simulink library "MedusaPremix"  (R2022b)
settings: Solver=VariableStepAuto  StartTime=0.0  StopTime=10.0  RelTol=1e-3
values from neighbouring files (symbols this model uses):
  PremixConfig = struct('sample_rate_in_hertz', sample_rate_in_hertz,                            'frame_size', frame_size,                            'rgain_SILENT_GAIN', rgain_SILENT_GAIN,                            'granularity', internal_granularity,                            'LR_in', LR_in, 'LR_out', LR_out,                            'CS_in', CS_in, 'CS_out', CS_out,                            'NumCenterOut' ...(+550 chars)    [MedusaPremixInit.m]
  PremixTune = MedusaPremixTuneInit(tuneFileName, headrestTuneFileName, overheadTuneFileName, MedusaParams)    [MedusaPremixInit.m]    (also in MedusaPremixTuneInit.m = load(tuneFileName))
undefined symbols (not defined in the file or in its folder): carModel, mode, MSConfig, Row
libraries: TuneVar x286, TOP x202, dspmtrx3 x146, FeaturePath x86, matrix_library x20, PooliirLib x8, Pooliir x4
(part 13 of 22)

== system MedusaPremix/Premix51/Full Mixing Matrix_Center Surround/Fader Downmix/Fading Forward ==
  backFadeGain : Inport
  forwardDownmixThreshold : Inport  Port=2
  forwardDownmixMax : Inport  Port=3
  Action Port : ActionPort
  Constant : Constant  OutDataTypeStr=single
  Divide : Product  Inputs=*/
  EPS : Constant  Value=eps('single')
  Max : MinMax  Function=max  Inputs=2
  Min : MinMax  Inputs=2
  Multiply : Product
  Subtract : Sum  Inputs=+-
  downmix : Outport  VectorParamsAs1DForOutWhenUnconnected=off
  wires:
  backFadeGain/1 -> Min/1
  forwardDownmixThreshold/1 -> Min/2, Max/1
  Constant/1 -> Subtract/1
  EPS/1 -> Max/2
  Min/1 -> Divide/1  "minFadeGain"
  Max/1 -> Divide/2
  Divide/1 -> Subtract/2
  Subtract/1 -> Multiply/1
  forwardDownmixMax/1 -> Multiply/2
  Multiply/1 -> downmix/1

== system MedusaPremix/Premix51/Full Mixing Matrix_Center Surround/Surround Level Control/Ramper ==
  RTC Recv Trigger : Inport
  target gains (linear) : Inport  Port=2
  ramp rate : Inport  Port=3
  ramp time : Inport  Port=4
  check sequence trigger : Inport  Port=5
  Data Store Memory : DataStoreMemory  DataStoreName=Premix_Freeze_CS  ReadBeforeWriteMsg=warning  WriteAfterWriteMsg=warning  WriteAfterReadMsg=warning  ShowAdditionalParam=off  OutDataTypeStr=boolean
  Data Store Memory1 : DataStoreMemory  DataStoreName=Premix_frameCount_CS  ReadBeforeWriteMsg=warning  WriteAfterWriteMsg=warning  WriteAfterReadMsg=warning  InitialValue=zeros(MedusaPremixConfig.CS_out,MedusaPremixConfig.CS_in)  ShowAdditionalParam=off  OutDataTypeStr=int32
  Data Store Memory2 : DataStoreMemory  DataStoreName=Premix_rampCoeff_CS  ReadBeforeWriteMsg=warning  WriteAfterWriteMsg=warning  WriteAfterReadMsg=warning  InitialValue=ones(MedusaPremixConfig.CS_out,MedusaPremixConfig.CS_in)  ShowAdditionalParam=off  OutDataTypeStr=single
  check sequence : MATLAB Function  TreatAsAtomicUnit=on
  control : MATLAB Function  TreatAsAtomicUnit=on
  process : MATLAB Function  TreatAsAtomicUnit=on
  ramping done : Outport  VectorParamsAs1DForOutWhenUnconnected=off
  wires:
  ramp time/1 -> control/3(rampTime)
  ramp rate/1 -> control/2(rampRate)
  check sequence trigger/1 -> check sequence/Trigger
  check sequence/1(done) -> ramping done/1
  RTC Recv Trigger/1 -> control/Trigger
  target gains (linear)/1 -> control/1(target_gains_linear)

== system MedusaPremix/Premix51/Full Mixing Matrix_Left/Fader Downmix/Fading Backward ==
  frontFadeGain : Inport
  backwardDownmixThreshold : Inport  Port=2
  backwardDownmixMax : Inport  Port=3
  Action Port : ActionPort
  Constant : Constant  OutDataTypeStr=single
  Divide : Product  Inputs=*/
  EPS : Constant  Value=eps('single')
  Max : MinMax  Function=max  Inputs=2
  Min : MinMax  Inputs=2
  Multiply : Product
  Subtract : Sum  Inputs=+-
  downmix : Outport  VectorParamsAs1DForOutWhenUnconnected=off
  wires:
  frontFadeGain/1 -> Min/1
  backwardDownmixThreshold/1 -> Min/2, Max/1
  Constant/1 -> Subtract/1
  EPS/1 -> Max/2
  Min/1 -> Divide/1  "minFadeGain"
  Max/1 -> Divide/2
  Divide/1 -> Subtract/2
  Subtract/1 -> Multiply/1
  backwardDownmixMax/1 -> Multiply/2
  Multiply/1 -> downmix/1

== system MedusaPremix/Premix51/Full Mixing Matrix_Left/Fader Downmix/Fading Forward ==
  backFadeGain : Inport
  forwardDownmixThreshold : Inport  Port=2
  forwardDownmixMax : Inport  Port=3
  Action Port : ActionPort
  Constant : Constant  OutDataTypeStr=single
  Divide : Product  Inputs=*/
  EPS : Constant  Value=eps('single')
  Max : MinMax  Function=max  Inputs=2
  Min : MinMax  Inputs=2
  Multiply : Product
  Subtract : Sum  Inputs=+-
  downmix : Outport  VectorParamsAs1DForOutWhenUnconnected=off
  wires:
  backFadeGain/1 -> Min/1
  forwardDownmixThreshold/1 -> Min/2, Max/1
  Constant/1 -> Subtract/1
  EPS/1 -> Max/2
  Min/1 -> Divide/1  "minFadeGain"
  Max/1 -> Divide/2
  Divide/1 -> Subtract/2
  Subtract/1 -> Multiply/1
  forwardDownmixMax/1 -> Multiply/2
  Multiply/1 -> downmix/1

== system MedusaPremix/Premix51/Full Mixing Matrix_Left/Surround Level Control/Ramper ==
  RTC Recv Trigger : Inport
  target gains (linear) : Inport  Port=2
  ramp rate : Inport  Port=3
  ramp time : Inport  Port=4
  check sequence trigger : Inport  Port=5
  Data Store Memory : DataStoreMemory  DataStoreName=Premix_Freeze_Left  ReadBeforeWriteMsg=warning  WriteAfterWriteMsg=warning  WriteAfterReadMsg=warning  ShowAdditionalParam=off  OutDataTypeStr=boolean
  Data Store Memory1 : DataStoreMemory  DataStoreName=Premix_frameCount_Left  ReadBeforeWriteMsg=warning  WriteAfterWriteMsg=warning  WriteAfterReadMsg=warning  InitialValue=zeros(MedusaPremixConfig.LR_out,MedusaPremixConfig.LR_in)  ShowAdditionalParam=off  OutDataTypeStr=int32
  Data Store Memory2 : DataStoreMemory  DataStoreName=Premix_rampCoeff_Left  ReadBeforeWriteMsg=warning  WriteAfterWriteMsg=warning  WriteAfterReadMsg=warning  InitialValue=ones(MedusaPremixConfig.LR_out,MedusaPremixConfig.LR_in)  ShowAdditionalParam=off  OutDataTypeStr=single
  check sequence : MATLAB Function  TreatAsAtomicUnit=on
  control : MATLAB Function  TreatAsAtomicUnit=on
  process : MATLAB Function  TreatAsAtomicUnit=on
  ramping done : Outport  VectorParamsAs1DForOutWhenUnconnected=off
  wires:
  ramp time/1 -> control/3(rampTime)
  ramp rate/1 -> control/2(rampRate)
  check sequence trigger/1 -> check sequence/Trigger
  check sequence/1(done) -> ramping done/1
  RTC Recv Trigger/1 -> control/Trigger
  target gains (linear)/1 -> control/1(target_gains_linear)

== system MedusaPremix/Premix51/Full Mixing Matrix_Right/Fader Downmix/Fading Backward ==
  frontFadeGain : Inport
  backwardDownmixThreshold : Inport  Port=2
  backwardDownmixMax : Inport  Port=3
  Action Port : ActionPort
  Constant : Constant  OutDataTypeStr=single
  Divide : Product  Inputs=*/
  EPS : Constant  Value=eps('single')
  Max : MinMax  Function=max  Inputs=2
  Min : MinMax  Inputs=2
  Multiply : Product
  Subtract : Sum  Inputs=+-
  downmix : Outport  VectorParamsAs1DForOutWhenUnconnected=off
  wires:
  frontFadeGain/1 -> Min/1
  backwardDownmixThreshold/1 -> Min/2, Max/1
  Constant/1 -> Subtract/1
  EPS/1 -> Max/2
  Min/1 -> Divide/1  "minFadeGain"
  Max/1 -> Divide/2
  Divide/1 -> Subtract/2
  Subtract/1 -> Multiply/1
  backwardDownmixMax/1 -> Multiply/2
  Multiply/1 -> downmix/1

== system MedusaPremix/Premix51/Full Mixing Matrix_Right/Fader Downmix/Fading Forward ==
  backFadeGain : Inport
  forwardDownmixThreshold : Inport  Port=2
  forwardDownmixMax : Inport  Port=3
  Action Port : ActionPort
  Constant : Constant  OutDataTypeStr=single
  Divide : Product  Inputs=*/
  EPS : Constant  Value=eps('single')
  Max : MinMax  Function=max  Inputs=2
  Min : MinMax  Inputs=2
  Multiply : Product
  Subtract : Sum  Inputs=+-
  downmix : Outport  VectorParamsAs1DForOutWhenUnconnected=off
  wires:
  backFadeGain/1 -> Min/1
  forwardDownmixThreshold/1 -> Min/2, Max/1
  Constant/1 -> Subtract/1
  EPS/1 -> Max/2
  Min/1 -> Divide/1  "minFadeGain"
  Max/1 -> Divide/2
  Divide/1 -> Subtract/2
  Subtract/1 -> Multiply/1
  forwardDownmixMax/1 -> Multiply/2
  Multiply/1 -> downmix/1

== system MedusaPremix/Premix51/Full Mixing Matrix_Right/Surround Level Control/Ramper ==
  RTC Recv Trigger : Inport
  target gains (linear) : Inport  Port=2
  ramp rate : Inport  Port=3
  ramp time : Inport  Port=4
  check sequence trigger : Inport  Port=5
  Data Store Memory : DataStoreMemory  DataStoreName=Premix_Freeze_Right  ReadBeforeWriteMsg=warning  WriteAfterWriteMsg=warning  WriteAfterReadMsg=warning  ShowAdditionalParam=off  OutDataTypeStr=boolean
  Data Store Memory1 : DataStoreMemory  DataStoreName=Premix_frameCount_Right  ReadBeforeWriteMsg=warning  WriteAfterWriteMsg=warning  WriteAfterReadMsg=warning  InitialValue=zeros(MedusaPremixConfig.LR_out,MedusaPremixConfig.LR_in)  ShowAdditionalParam=off  OutDataTypeStr=int32
  Data Store Memory2 : DataStoreMemory  DataStoreName=Premix_rampCoeff_Right  ReadBeforeWriteMsg=warning  WriteAfterWriteMsg=warning  WriteAfterReadMsg=warning  InitialValue=ones(MedusaPremixConfig.LR_out,MedusaPremixConfig.LR_in)  ShowAdditionalParam=off  OutDataTypeStr=single
  check sequence : MATLAB Function  TreatAsAtomicUnit=on
  control : MATLAB Function  TreatAsAtomicUnit=on
  process : MATLAB Function  TreatAsAtomicUnit=on
  ramping done : Outport  VectorParamsAs1DForOutWhenUnconnected=off
  wires:
  ramp time/1 -> control/3(rampTime)
  ramp rate/1 -> control/2(rampRate)
  check sequence trigger/1 -> check sequence/Trigger
  check sequence/1(done) -> ramping done/1
  RTC Recv Trigger/1 -> control/Trigger
  target gains (linear)/1 -> control/1(target_gains_linear)

== system MedusaPremix/Premix51WithMonoSurround/CS Processing/Mono-Surround/Left Mixer ==
  AudioIn : Inport
  MixCoeff : Inport  Port=2
  Matrix Multiply1 : Product  Multiplication=Matrix(*)
  Transpose1 : Math  Operator=transpose  SignedPower=on
  Output : Outport  VectorParamsAs1DForOutWhenUnconnected=off
  wires:
  Matrix Multiply1/1 -> Output/1
  AudioIn/1 -> Matrix Multiply1/1
  MixCoeff/1 -> Transpose1/1
  Transpose1/1 -> Matrix Multiply1/2

== system MedusaPremix/Premix51WithMonoSurround/CS Processing/Mono-Surround/MS Tune ==
  TOP : TOP/TOP  TriggerInit=[260 -150 405 -90]  TopName=Phi  DataType=single  BankNumber=0  Role=Automatic
      settings: SourceProductName=Bose Talaria
  TOP1 : TOP/TOP  TriggerInit=[260 -70 405 -10]  TopName=CosPhi  DataType=single  BankNumber=0  Role=Automatic
      settings: SourceProductName=Bose Talaria
  TOP2 : TOP/TOP  TriggerInit=[260 10 405 70]  TopName=SinPhi  DataType=single  BankNumber=0  Role=Automatic
      settings: SourceProductName=Bose Talaria
  TranslateTrigger : TuneVar/TranslateTrigger  TriggerInit=[66 -245 104 -190]
      settings: SourceProductName=Bose Talaria
  Tune Variable : TuneVar/Tune Variable  TuneName=PhaseAngle  SpecifyMaxSize=off  VariableDim=1 (Row)  MaxSize=[1 1]  PackageName=mode  TunabilityNumber=1  MinValue=[]  MaxValue=[]  TriggerInit=[-270 -65 -100 -15]  MaskValue=MSConfig.DefaultPhaseAngle
      settings: SourceProductName=Bose Talaria
  translation : MATLAB Function  TreatAsAtomicUnit=on
  phi : Outport  VectorParamsAs1DForOutWhenUnconnected=off
  cos(phi) : Outport  Port=2  VectorParamsAs1DForOutWhenUnconnected=off
  sin(phi) : Outport  Port=3  VectorParamsAs1DForOutWhenUnconnected=off
  wires:
  translation/1(phi) -> TOP/1
  TranslateTrigger/1 -> translation/Trigger
  TOP/1 -> phi/1  "Phi"
  Tune Variable/1 -> translation/1(PhaseAngle)  "PhaseAngle"
  translation/2(cos_phi) -> TOP1/1
  TOP1/1 -> cos(phi)/1  "CosPhi"
  translation/3(sin_phi) -> TOP2/1
  TOP2/1 -> sin(phi)/1  "SinPhi"

== system MedusaPremix/Premix51WithMonoSurround/CS Processing/Mono-Surround/Right Mixer ==
  AudioIn : Inport
  MixCoeff : Inport  Port=2
  Matrix Multiply1 : Product  Multiplication=Matrix(*)
  Transpose1 : Math  Operator=transpose  SignedPower=on
  Output : Outport  VectorParamsAs1DForOutWhenUnconnected=off
  wires:
  Matrix Multiply1/1 -> Output/1
  AudioIn/1 -> Matrix Multiply1/1
  MixCoeff/1 -> Transpose1/1
  Transpose1/1 -> Matrix Multiply1/2

== system MedusaPremix/Premix51WithMonoSurround/CS Processing/Mono-Surround/Right Mixer1 ==
  AudioIn : Inport
  MixCoeff : Inport  Port=2
  Matrix Multiply1 : Product  Multiplication=Matrix(*)
  Transpose1 : Math  Operator=transpose  SignedPower=on
  Output : Outport  VectorParamsAs1DForOutWhenUnconnected=off
  wires:
  Matrix Multiply1/1 -> Output/1
  AudioIn/1 -> Matrix Multiply1/1
  MixCoeff/1 -> Transpose1/1
  Transpose1/1 -> Matrix Multiply1/2

== system MedusaPremix/Premix51WithMonoSurround/CS Processing/Mono-Surround/SOS A ==
  AudioIn : Inport
  TuneIn : Inport  Port=2
  Hilbert SOS A : Subsystem  TreatAsAtomicUnit=on
  If : If  IfExpression=(u1==0) | (u1==180)
  Merge : Merge
  Pass-through : Subsystem  TreatAsAtomicUnit=on
  Out : Outport  VectorParamsAs1DForOutWhenUnconnected=off
  wires:
  AudioIn/1 -> Hilbert SOS A/1(AudioIn), Pass-through/1(In1)
  If/1 -> Pass-through/Action
  If/2 -> Hilbert SOS A/Action
  TuneIn/1 -> If/1
  Pass-through/1(Out1) -> Merge/1
  Hilbert SOS A/1(Out) -> Merge/2
  Merge/1 -> Out/1

== system MedusaPremix/Premix51WithMonoSurround/CS Processing/Mono-Surround/SOS B ==
  AudioIn : Inport
  TuneIn : Inport  Port=2
  Hilbert SOS B : Subsystem  TreatAsAtomicUnit=on
  If : If  IfExpression=(u1==0) | (u1==180)
  Merge : Merge
  Pass-through : Subsystem  TreatAsAtomicUnit=on
  Out : Outport  VectorParamsAs1DForOutWhenUnconnected=off
  wires:
  AudioIn/1 -> Hilbert SOS B/1(AudioIn), Pass-through/1(In1)
  If/1 -> Pass-through/Action
  If/2 -> Hilbert SOS B/Action
  TuneIn/1 -> If/1
  Pass-through/1(Out1) -> Merge/1
  Hilbert SOS B/1(Out) -> Merge/2
  Merge/1 -> Out/1

== system MedusaPremix/Premix51WithMonoSurround/Full Mixing Matrix_Center Surround/Fader Downmix/Fading Backward ==
  frontFadeGain : Inport
  backwardDownmixThreshold : Inport  Port=2
  backwardDownmixMax : Inport  Port=3
  Action Port : ActionPort
  Constant : Constant  OutDataTypeStr=single
  Divide : Product  Inputs=*/
  EPS : Constant  Value=eps('single')
  Max : MinMax  Function=max  Inputs=2
  Min : MinMax  Inputs=2
  Multiply : Product
  Subtract : Sum  Inputs=+-
  downmix : Outport  VectorParamsAs1DForOutWhenUnconnected=off
  wires:
  frontFadeGain/1 -> Min/1
  backwardDownmixThreshold/1 -> Min/2, Max/1
  Constant/1 -> Subtract/1
  EPS/1 -> Max/2
  Min/1 -> Divide/1  "minFadeGain"
  Max/1 -> Divide/2
  Divide/1 -> Subtract/2
  Subtract/1 -> Multiply/1
  backwardDownmixMax/1 -> Multiply/2
  Multiply/1 -> downmix/1

== system MedusaPremix/Premix51WithMonoSurround/Full Mixing Matrix_Center Surround/Fader Downmix/Fading Forward ==
  backFadeGain : Inport
  forwardDownmixThreshold : Inport  Port=2
  forwardDownmixMax : Inport  Port=3
  Action Port : ActionPort
  Constant : Constant  OutDataTypeStr=single
  Divide : Product  Inputs=*/
  EPS : Constant  Value=eps('single')
  Max : MinMax  Function=max  Inputs=2
  Min : MinMax  Inputs=2
  Multiply : Product
  Subtract : Sum  Inputs=+-
  downmix : Outport  VectorParamsAs1DForOutWhenUnconnected=off
  wires:
  backFadeGain/1 -> Min/1
  forwardDownmixThreshold/1 -> Min/2, Max/1
  Constant/1 -> Subtract/1
  EPS/1 -> Max/2
  Min/1 -> Divide/1  "minFadeGain"
  Max/1 -> Divide/2
  Divide/1 -> Subtract/2
  Subtract/1 -> Multiply/1
  forwardDownmixMax/1 -> Multiply/2
  Multiply/1 -> downmix/1

== system MedusaPremix/Premix51WithMonoSurround/Full Mixing Matrix_Center Surround/Surround Level Control/Ramper ==
  RTC Recv Trigger : Inport
  target gains (linear) : Inport  Port=2
  ramp rate : Inport  Port=3
  ramp time : Inport  Port=4
  check sequence trigger : Inport  Port=5
  Data Store Memory : DataStoreMemory  DataStoreName=Premix_Freeze_CS  ReadBeforeWriteMsg=warning  WriteAfterWriteMsg=warning  WriteAfterReadMsg=warning  ShowAdditionalParam=off  OutDataTypeStr=boolean
  Data Store Memory1 : DataStoreMemory  DataStoreName=Premix_frameCount_CS  ReadBeforeWriteMsg=warning  WriteAfterWriteMsg=warning  WriteAfterReadMsg=warning  InitialValue=zeros(MedusaPremixConfig.CS_out,MedusaPremixConfig.CS_in)  ShowAdditionalParam=off  OutDataTypeStr=int32
  Data Store Memory2 : DataStoreMemory  DataStoreName=Premix_rampCoeff_CS  ReadBeforeWriteMsg=warning  WriteAfterWriteMsg=warning  WriteAfterReadMsg=warning  InitialValue=ones(MedusaPremixConfig.CS_out,MedusaPremixConfig.CS_in)  ShowAdditionalParam=off  OutDataTypeStr=single
  check sequence : MATLAB Function  TreatAsAtomicUnit=on
  control : MATLAB Function  TreatAsAtomicUnit=on
  process : MATLAB Function  TreatAsAtomicUnit=on
  ramping done : Outport  VectorParamsAs1DForOutWhenUnconnected=off
  wires:
  ramp time/1 -> control/3(rampTime)
  ramp rate/1 -> control/2(rampRate)
  check sequence trigger/1 -> check sequence/Trigger
  check sequence/1(done) -> ramping done/1
  RTC Recv Trigger/1 -> control/Trigger
  target gains (linear)/1 -> control/1(target_gains_linear)

== system MedusaPremix/Premix51WithMonoSurround/Full Mixing Matrix_Left/Fader Downmix/Fading Backward ==
  frontFadeGain : Inport
  backwardDownmixThreshold : Inport  Port=2
  backwardDownmixMax : Inport  Port=3
  Action Port : ActionPort
  Constant : Constant  OutDataTypeStr=single
  Divide : Product  Inputs=*/
  EPS : Constant  Value=eps('single')
  Max : MinMax  Function=max  Inputs=2
  Min : MinMax  Inputs=2
  Multiply : Product
  Subtract : Sum  Inputs=+-
  downmix : Outport  VectorParamsAs1DForOutWhenUnconnected=off
  wires:
  frontFadeGain/1 -> Min/1
  backwardDownmixThreshold/1 -> Min/2, Max/1
  Constant/1 -> Subtract/1
  EPS/1 -> Max/2
  Min/1 -> Divide/1  "minFadeGain"
  Max/1 -> Divide/2
  Divide/1 -> Subtract/2
  Subtract/1 -> Multiply/1
  backwardDownmixMax/1 -> Multiply/2
  Multiply/1 -> downmix/1

== system MedusaPremix/Premix51WithMonoSurround/Full Mixing Matrix_Left/Fader Downmix/Fading Forward ==
  backFadeGain : Inport
  forwardDownmixThreshold : Inport  Port=2
  forwardDownmixMax : Inport  Port=3
  Action Port : ActionPort
  Constant : Constant  OutDataTypeStr=single
  Divide : Product  Inputs=*/
  EPS : Constant  Value=eps('single')
  Max : MinMax  Function=max  Inputs=2
  Min : MinMax  Inputs=2
  Multiply : Product
  Subtract : Sum  Inputs=+-
  downmix : Outport  VectorParamsAs1DForOutWhenUnconnected=off
  wires:
  backFadeGain/1 -> Min/1
  forwardDownmixThreshold/1 -> Min/2, Max/1
  Constant/1 -> Subtract/1
  EPS/1 -> Max/2
  Min/1 -> Divide/1  "minFadeGain"
  Max/1 -> Divide/2
  Divide/1 -> Subtract/2
  Subtract/1 -> Multiply/1
  forwardDownmixMax/1 -> Multiply/2
  Multiply/1 -> downmix/1

== system MedusaPremix/Premix51WithMonoSurround/Full Mixing Matrix_Left/Surround Level Control/Ramper ==
  RTC Recv Trigger : Inport
  target gains (linear) : Inport  Port=2
  ramp rate : Inport  Port=3
  ramp time : Inport  Port=4
  check sequence trigger : Inport  Port=5
  Data Store Memory : DataStoreMemory  DataStoreName=Premix_Freeze_Left  ReadBeforeWriteMsg=warning  WriteAfterWriteMsg=warning  WriteAfterReadMsg=warning  ShowAdditionalParam=off  OutDataTypeStr=boolean
  Data Store Memory1 : DataStoreMemory  DataStoreName=Premix_frameCount_Left  ReadBeforeWriteMsg=warning  WriteAfterWriteMsg=warning  WriteAfterReadMsg=warning  InitialValue=zeros(MedusaPremixConfig.LR_out,MedusaPremixConfig.LR_in)  ShowAdditionalParam=off  OutDataTypeStr=int32
  Data Store Memory2 : DataStoreMemory  DataStoreName=Premix_rampCoeff_Left  ReadBeforeWriteMsg=warning  WriteAfterWriteMsg=warning  WriteAfterReadMsg=warning  InitialValue=ones(MedusaPremixConfig.LR_out,MedusaPremixConfig.LR_in)  ShowAdditionalParam=off  OutDataTypeStr=single
  check sequence : MATLAB Function  TreatAsAtomicUnit=on
  control : MATLAB Function  TreatAsAtomicUnit=on
  process : MATLAB Function  TreatAsAtomicUnit=on
  ramping done : Outport  VectorParamsAs1DForOutWhenUnconnected=off
  wires:
  ramp time/1 -> control/3(rampTime)
  ramp rate/1 -> control/2(rampRate)
  check sequence trigger/1 -> check sequence/Trigger
  check sequence/1(done) -> ramping done/1
  RTC Recv Trigger/1 -> control/Trigger
  target gains (linear)/1 -> control/1(target_gains_linear)

== system MedusaPremix/Premix51WithMonoSurround/Full Mixing Matrix_Right/Fader Downmix/Fading Backward ==
  frontFadeGain : Inport
  backwardDownmixThreshold : Inport  Port=2
  backwardDownmixMax : Inport  Port=3
  Action Port : ActionPort
  Constant : Constant  OutDataTypeStr=single
  Divide : Product  Inputs=*/
  EPS : Constant  Value=eps('single')
  Max : MinMax  Function=max  Inputs=2
  Min : MinMax  Inputs=2
  Multiply : Product
  Subtract : Sum  Inputs=+-
  downmix : Outport  VectorParamsAs1DForOutWhenUnconnected=off
  wires:
  frontFadeGain/1 -> Min/1
  backwardDownmixThreshold/1 -> Min/2, Max/1
  Constant/1 -> Subtract/1
  EPS/1 -> Max/2
  Min/1 -> Divide/1  "minFadeGain"
  Max/1 -> Divide/2
  Divide/1 -> Subtract/2
  Subtract/1 -> Multiply/1
  backwardDownmixMax/1 -> Multiply/2
  Multiply/1 -> downmix/1

== system MedusaPremix/Premix51WithMonoSurround/Full Mixing Matrix_Right/Fader Downmix/Fading Forward ==
  backFadeGain : Inport
  forwardDownmixThreshold : Inport  Port=2
  forwardDownmixMax : Inport  Port=3
  Action Port : ActionPort
  Constant : Constant  OutDataTypeStr=single
  Divide : Product  Inputs=*/
  EPS : Constant  Value=eps('single')
  Max : MinMax  Function=max  Inputs=2
  Min : MinMax  Inputs=2
  Multiply : Product
  Subtract : Sum  Inputs=+-
  downmix : Outport  VectorParamsAs1DForOutWhenUnconnected=off
  wires:
  backFadeGain/1 -> Min/1
  forwardDownmixThreshold/1 -> Min/2, Max/1
  Constant/1 -> Subtract/1
  EPS/1 -> Max/2
  Min/1 -> Divide/1  "minFadeGain"
  Max/1 -> Divide/2
  Divide/1 -> Subtract/2
  Subtract/1 -> Multiply/1
  forwardDownmixMax/1 -> Multiply/2
  Multiply/1 -> downmix/1

== system MedusaPremix/Premix51WithMonoSurround/Full Mixing Matrix_Right/Surround Level Control/Ramper ==
  RTC Recv Trigger : Inport
  target gains (linear) : Inport  Port=2
  ramp rate : Inport  Port=3
  ramp time : Inport  Port=4
  check sequence trigger : Inport  Port=5
  Data Store Memory : DataStoreMemory  DataStoreName=Premix_Freeze_Right  ReadBeforeWriteMsg=warning  WriteAfterWriteMsg=warning  WriteAfterReadMsg=warning  ShowAdditionalParam=off  OutDataTypeStr=boolean
  Data Store Memory1 : DataStoreMemory  DataStoreName=Premix_frameCount_Right  ReadBeforeWriteMsg=warning  WriteAfterWriteMsg=warning  WriteAfterReadMsg=warning  InitialValue=zeros(MedusaPremixConfig.LR_out,MedusaPremixConfig.LR_in)  ShowAdditionalParam=off  OutDataTypeStr=int32
  Data Store Memory2 : DataStoreMemory  DataStoreName=Premix_rampCoeff_Right  ReadBeforeWriteMsg=warning  WriteAfterWriteMsg=warning  WriteAfterReadMsg=warning  InitialValue=ones(MedusaPremixConfig.LR_out,MedusaPremixConfig.LR_in)  ShowAdditionalParam=off  OutDataTypeStr=single
  check sequence : MATLAB Function  TreatAsAtomicUnit=on
  control : MATLAB Function  TreatAsAtomicUnit=on
  process : MATLAB Function  TreatAsAtomicUnit=on
  ramping done : Outport  VectorParamsAs1DForOutWhenUnconnected=off
  wires:
  ramp time/1 -> control/3(rampTime)
  ramp rate/1 -> control/2(rampRate)
  check sequence trigger/1 -> check sequence/Trigger
  check sequence/1(done) -> ramping done/1
  RTC Recv Trigger/1 -> control/Trigger
  target gains (linear)/1 -> control/1(target_gains_linear)

== system MedusaPremix/Premix51WithMonoSurroundAndCae/CS Processing/Mono-Surround/Left Mixer ==
  AudioIn : Inport
  MixCoeff : Inport  Port=2
  Matrix Multiply1 : Product  Multiplication=Matrix(*)
  Transpose1 : Math  Operator=transpose  SignedPower=on
  Output : Outport  VectorParamsAs1DForOutWhenUnconnected=off
  wires:
  Matrix Multiply1/1 -> Output/1
  AudioIn/1 -> Matrix Multiply1/1
  MixCoeff/1 -> Transpose1/1
  Transpose1/1 -> Matrix Multiply1/2

== system MedusaPremix/Premix51WithMonoSurroundAndCae/CS Processing/Mono-Surround/MS Tune ==
  TOP : TOP/TOP  TriggerInit=[260 -150 405 -90]  TopName=Phi  DataType=single  BankNumber=0  Role=Automatic
      settings: SourceProductName=Bose Talaria
  TOP1 : TOP/TOP  TriggerInit=[260 -70 405 -10]  TopName=CosPhi  DataType=single  BankNumber=0  Role=Automatic
      settings: SourceProductName=Bose Talaria
  TOP2 : TOP/TOP  TriggerInit=[260 10 405 70]  TopName=SinPhi  DataType=single  BankNumber=0  Role=Automatic
      settings: SourceProductName=Bose Talaria
  TranslateTrigger : TuneVar/TranslateTrigger  TriggerInit=[66 -245 104 -190]
      settings: SourceProductName=Bose Talaria
  Tune Variable : TuneVar/Tune Variable  TuneName=PhaseAngle  SpecifyMaxSize=off  VariableDim=1 (Row)  MaxSize=[1 1]  PackageName=mode  TunabilityNumber=1  MinValue=[]  MaxValue=[]  TriggerInit=[-270 -65 -100 -15]  MaskValue=MSConfig.DefaultPhaseAngle
      settings: SourceProductName=Bose Talaria
  translation : MATLAB Function  TreatAsAtomicUnit=on
  phi : Outport  VectorParamsAs1DForOutWhenUnconnected=off
  cos(phi) : Outport  Port=2  VectorParamsAs1DForOutWhenUnconnected=off
  sin(phi) : Outport  Port=3  VectorParamsAs1DForOutWhenUnconnected=off
  wires:
  translation/1(phi) -> TOP/1
  TranslateTrigger/1 -> translation/Trigger
  TOP/1 -> phi/1  "Phi"
  Tune Variable/1 -> translation/1(PhaseAngle)  "PhaseAngle"
  translation/2(cos_phi) -> TOP1/1
  TOP1/1 -> cos(phi)/1  "CosPhi"
  translation/3(sin_phi) -> TOP2/1
  TOP2/1 -> sin(phi)/1  "SinPhi"

== system MedusaPremix/Premix51WithMonoSurroundAndCae/CS Processing/Mono-Surround/Right Mixer ==
  AudioIn : Inport
  MixCoeff : Inport  Port=2
  Matrix Multiply1 : Product  Multiplication=Matrix(*)
  Transpose1 : Math  Operator=transpose  SignedPower=on
  Output : Outport  VectorParamsAs1DForOutWhenUnconnected=off
  wires:
  Matrix Multiply1/1 -> Output/1
  AudioIn/1 -> Matrix Multiply1/1
  MixCoeff/1 -> Transpose1/1
  Transpose1/1 -> Matrix Multiply1/2

== system MedusaPremix/Premix51WithMonoSurroundAndCae/CS Processing/Mono-Surround/Right Mixer1 ==
  AudioIn : Inport
  MixCoeff : Inport  Port=2
  Matrix Multiply1 : Product  Multiplication=Matrix(*)
  Transpose1 : Math  Operator=transpose  SignedPower=on
  Output : Outport  VectorParamsAs1DForOutWhenUnconnected=off
  wires:
  Matrix Multiply1/1 -> Output/1
  AudioIn/1 -> Matrix Multiply1/1
  MixCoeff/1 -> Transpose1/1
  Transpose1/1 -> Matrix Multiply1/2

== system MedusaPremix/Premix51WithMonoSurroundAndCae/CS Processing/Mono-Surround/SOS A ==
  AudioIn : Inport
  TuneIn : Inport  Port=2
  Hilbert SOS A : Subsystem  TreatAsAtomicUnit=on
  If : If  IfExpression=(u1==0) | (u1==180)
  Merge : Merge
  Pass-through : Subsystem  TreatAsAtomicUnit=on
  Out : Outport  VectorParamsAs1DForOutWhenUnconnected=off
  wires:
  AudioIn/1 -> Hilbert SOS A/1(AudioIn), Pass-through/1(In1)
  If/1 -> Pass-through/Action
  If/2 -> Hilbert SOS A/Action
  TuneIn/1 -> If/1
  Pass-through/1(Out1) -> Merge/1
  Hilbert SOS A/1(Out) -> Merge/2
  Merge/1 -> Out/1

== system MedusaPremix/Premix51WithMonoSurroundAndCae/CS Processing/Mono-Surround/SOS B ==
  AudioIn : Inport
  TuneIn : Inport  Port=2
  Hilbert SOS B : Subsystem  TreatAsAtomicUnit=on
  If : If  IfExpression=(u1==0) | (u1==180)
  Merge : Merge
  Pass-through : Subsystem  TreatAsAtomicUnit=on
  Out : Outport  VectorParamsAs1DForOutWhenUnconnected=off
  wires:
  AudioIn/1 -> Hilbert SOS B/1(AudioIn), Pass-through/1(In1)
  If/1 -> Pass-through/Action
  If/2 -> Hilbert SOS B/Action
  TuneIn/1 -> If/1
  Pass-through/1(Out1) -> Merge/1
  Hilbert SOS B/1(Out) -> Merge/2
  Merge/1 -> Out/1

== system MedusaPremix/Premix51WithMonoSurroundAndCae/Full Mixing Matrix_Center Surround/Fader Downmix/Fading Backward ==
  frontFadeGain : Inport
  backwardDownmixThreshold : Inport  Port=2
  backwardDownmixMax : Inport  Port=3
  Action Port : ActionPort
  Constant : Constant  OutDataTypeStr=single
  Divide : Product  Inputs=*/
  EPS : Constant  Value=eps('single')
  Max : MinMax  Function=max  Inputs=2
  Min : MinMax  Inputs=2
  Multiply : Product
  Subtract : Sum  Inputs=+-
  downmix : Outport  VectorParamsAs1DForOutWhenUnconnected=off
  wires:
  Multiply/1 -> downmix/1
  backwardDownmixMax/1 -> Multiply/2
  Subtract/1 -> Multiply/1
  Divide/1 -> Subtract/2
  Max/1 -> Divide/2
  Min/1 -> Divide/1  "minFadeGain"
  EPS/1 -> Max/2
  Constant/1 -> Subtract/1
  backwardDownmixThreshold/1 -> Max/1, Min/2
  frontFadeGain/1 -> Min/1

== system MedusaPremix/Premix51WithMonoSurroundAndCae/Full Mixing Matrix_Center Surround/Fader Downmix/Fading Forward ==
  backFadeGain : Inport
  forwardDownmixThreshold : Inport  Port=2
  forwardDownmixMax : Inport  Port=3
  Action Port : ActionPort
  Constant : Constant  OutDataTypeStr=single
  Divide : Product  Inputs=*/
  EPS : Constant  Value=eps('single')
  Max : MinMax  Function=max  Inputs=2
  Min : MinMax  Inputs=2
  Multiply : Product
  Subtract : Sum  Inputs=+-
  downmix : Outport  VectorParamsAs1DForOutWhenUnconnected=off
  wires:
  Multiply/1 -> downmix/1
  forwardDownmixMax/1 -> Multiply/2
  Subtract/1 -> Multiply/1
  Divide/1 -> Subtract/2
  Max/1 -> Divide/2
  Min/1 -> Divide/1  "minFadeGain"
  EPS/1 -> Max/2
  Constant/1 -> Subtract/1
  forwardDownmixThreshold/1 -> Max/1, Min/2
  backFadeGain/1 -> Min/1

== system MedusaPremix/Premix51WithMonoSurroundAndCae/Full Mixing Matrix_Center Surround/Surround Level Control/Ramper ==
  RTC Recv Trigger : Inport
  target gains (linear) : Inport  Port=2
  ramp rate : Inport  Port=3
  ramp time : Inport  Port=4
  check sequence trigger : Inport  Port=5
  Data Store Memory : DataStoreMemory  DataStoreName=Premix_Freeze_CS  ReadBeforeWriteMsg=warning  WriteAfterWriteMsg=warning  WriteAfterReadMsg=warning  ShowAdditionalParam=off  OutDataTypeStr=boolean
  Data Store Memory1 : DataStoreMemory  DataStoreName=Premix_frameCount_CS  ReadBeforeWriteMsg=warning  WriteAfterWriteMsg=warning  WriteAfterReadMsg=warning  InitialValue=zeros(MedusaPremixConfig.CS_out,MedusaPremixConfig.CS_in)  ShowAdditionalParam=off  OutDataTypeStr=int32
  Data Store Memory2 : DataStoreMemory  DataStoreName=Premix_rampCoeff_CS  ReadBeforeWriteMsg=warning  WriteAfterWriteMsg=warning  WriteAfterReadMsg=warning  InitialValue=ones(MedusaPremixConfig.CS_out,MedusaPremixConfig.CS_in)  ShowAdditionalParam=off  OutDataTypeStr=single
  check sequence : MATLAB Function  TreatAsAtomicUnit=on
  control : MATLAB Function  TreatAsAtomicUnit=on
  process : MATLAB Function  TreatAsAtomicUnit=on
  ramping done : Outport  VectorParamsAs1DForOutWhenUnconnected=off
  wires:
  target gains (linear)/1 -> control/1(target_gains_linear)
  RTC Recv Trigger/1 -> control/Trigger
  check sequence/1(done) -> ramping done/1
  check sequence trigger/1 -> check sequence/Trigger
  ramp rate/1 -> control/2(rampRate)
  ramp time/1 -> control/3(rampTime)

== system MedusaPremix/Premix51WithMonoSurroundAndCae/Full Mixing Matrix_Left/Fader Downmix/Fading Backward ==
  frontFadeGain : Inport
  backwardDownmixThreshold : Inport  Port=2
  backwardDownmixMax : Inport  Port=3
  Action Port : ActionPort
  Constant : Constant  OutDataTypeStr=single
  Divide : Product  Inputs=*/
  EPS : Constant  Value=eps('single')
  Max : MinMax  Function=max  Inputs=2
  Min : MinMax  Inputs=2
  Multiply : Product
  Subtract : Sum  Inputs=+-
  downmix : Outport  VectorParamsAs1DForOutWhenUnconnected=off
  wires:
  Multiply/1 -> downmix/1
  backwardDownmixMax/1 -> Multiply/2
  Subtract/1 -> Multiply/1
  Divide/1 -> Subtract/2
  Max/1 -> Divide/2
  Min/1 -> Divide/1  "minFadeGain"
  EPS/1 -> Max/2
  Constant/1 -> Subtract/1
  backwardDownmixThreshold/1 -> Max/1, Min/2
  frontFadeGain/1 -> Min/1

== system MedusaPremix/Premix51WithMonoSurroundAndCae/Full Mixing Matrix_Left/Fader Downmix/Fading Forward ==
  backFadeGain : Inport
  forwardDownmixThreshold : Inport  Port=2
  forwardDownmixMax : Inport  Port=3
  Action Port : ActionPort
  Constant : Constant  OutDataTypeStr=single
  Divide : Product  Inputs=*/
  EPS : Constant  Value=eps('single')
  Max : MinMax  Function=max  Inputs=2
  Min : MinMax  Inputs=2
  Multiply : Product
  Subtract : Sum  Inputs=+-
  downmix : Outport  VectorParamsAs1DForOutWhenUnconnected=off
  wires:
  Multiply/1 -> downmix/1
  forwardDownmixMax/1 -> Multiply/2
  Subtract/1 -> Multiply/1
  Divide/1 -> Subtract/2
  Max/1 -> Divide/2
  Min/1 -> Divide/1  "minFadeGain"
  EPS/1 -> Max/2
  Constant/1 -> Subtract/1
  forwardDownmixThreshold/1 -> Max/1, Min/2
  backFadeGain/1 -> Min/1

== system MedusaPremix/Premix51WithMonoSurroundAndCae/Full Mixing Matrix_Left/Surround Level Control/Ramper ==
  RTC Recv Trigger : Inport
  target gains (linear) : Inport  Port=2
  ramp rate : Inport  Port=3
  ramp time : Inport  Port=4
  check sequence trigger : Inport  Port=5
  Data Store Memory : DataStoreMemory  DataStoreName=Premix_Freeze_Left  ReadBeforeWriteMsg=warning  WriteAfterWriteMsg=warning  WriteAfterReadMsg=warning  ShowAdditionalParam=off  OutDataTypeStr=boolean
  Data Store Memory1 : DataStoreMemory  DataStoreName=Premix_frameCount_Left  ReadBeforeWriteMsg=warning  WriteAfterWriteMsg=warning  WriteAfterReadMsg=warning  InitialValue=zeros(MedusaPremixConfig.LR_out,MedusaPremixConfig.LR_in)  ShowAdditionalParam=off  OutDataTypeStr=int32
  Data Store Memory2 : DataStoreMemory  DataStoreName=Premix_rampCoeff_Left  ReadBeforeWriteMsg=warning  WriteAfterWriteMsg=warning  WriteAfterReadMsg=warning  InitialValue=ones(MedusaPremixConfig.LR_out,MedusaPremixConfig.LR_in)  ShowAdditionalParam=off  OutDataTypeStr=single
  check sequence : MATLAB Function  TreatAsAtomicUnit=on
  control : MATLAB Function  TreatAsAtomicUnit=on
  process : MATLAB Function  TreatAsAtomicUnit=on
  ramping done : Outport  VectorParamsAs1DForOutWhenUnconnected=off
  wires:
  target gains (linear)/1 -> control/1(target_gains_linear)
  RTC Recv Trigger/1 -> control/Trigger
  check sequence/1(done) -> ramping done/1
  check sequence trigger/1 -> check sequence/Trigger
  ramp time/1 -> control/3(rampTime)
  ramp rate/1 -> control/2(rampRate)

== system MedusaPremix/Premix51WithMonoSurroundAndCae/Full Mixing Matrix_Right/Fader Downmix/Fading Backward ==
  frontFadeGain : Inport
  backwardDownmixThreshold : Inport  Port=2
  backwardDownmixMax : Inport  Port=3
  Action Port : ActionPort
  Constant : Constant  OutDataTypeStr=single
  Divide : Product  Inputs=*/
  EPS : Constant  Value=eps('single')
  Max : MinMax  Function=max  Inputs=2
  Min : MinMax  Inputs=2
  Multiply : Product
  Subtract : Sum  Inputs=+-
  downmix : Outport  VectorParamsAs1DForOutWhenUnconnected=off
  wires:
  Multiply/1 -> downmix/1
  backwardDownmixMax/1 -> Multiply/2
  Subtract/1 -> Multiply/1
  Divide/1 -> Subtract/2
  Max/1 -> Divide/2
  Min/1 -> Divide/1  "minFadeGain"
  EPS/1 -> Max/2
  Constant/1 -> Subtract/1
  backwardDownmixThreshold/1 -> Max/1, Min/2
  frontFadeGain/1 -> Min/1

== system MedusaPremix/Premix51WithMonoSurroundAndCae/Full Mixing Matrix_Right/Fader Downmix/Fading Forward ==
  backFadeGain : Inport
  forwardDownmixThreshold : Inport  Port=2
  forwardDownmixMax : Inport  Port=3
  Action Port : ActionPort
  Constant : Constant  OutDataTypeStr=single
  Divide : Product  Inputs=*/
  EPS : Constant  Value=eps('single')
  Max : MinMax  Function=max  Inputs=2
  Min : MinMax  Inputs=2
  Multiply : Product
  Subtract : Sum  Inputs=+-
  downmix : Outport  VectorParamsAs1DForOutWhenUnconnected=off
  wires:
  Multiply/1 -> downmix/1
  forwardDownmixMax/1 -> Multiply/2
  Subtract/1 -> Multiply/1
  Divide/1 -> Subtract/2
  Max/1 -> Divide/2
  Min/1 -> Divide/1  "minFadeGain"
  EPS/1 -> Max/2
  Constant/1 -> Subtract/1
  forwardDownmixThreshold/1 -> Max/1, Min/2
  backFadeGain/1 -> Min/1

== system MedusaPremix/Premix51WithMonoSurroundAndCae/Full Mixing Matrix_Right/Surround Level Control/Ramper ==
  RTC Recv Trigger : Inport
  target gains (linear) : Inport  Port=2
  ramp rate : Inport  Port=3
  ramp time : Inport  Port=4
  check sequence trigger : Inport  Port=5
  Data Store Memory : DataStoreMemory  DataStoreName=Premix_Freeze_Right  ReadBeforeWriteMsg=warning  WriteAfterWriteMsg=warning  WriteAfterReadMsg=warning  ShowAdditionalParam=off  OutDataTypeStr=boolean
  Data Store Memory1 : DataStoreMemory  DataStoreName=Premix_frameCount_Right  ReadBeforeWriteMsg=warning  WriteAfterWriteMsg=warning  WriteAfterReadMsg=warning  InitialValue=zeros(MedusaPremixConfig.LR_out,MedusaPremixConfig.LR_in)  ShowAdditionalParam=off  OutDataTypeStr=int32
  Data Store Memory2 : DataStoreMemory  DataStoreName=Premix_rampCoeff_Right  ReadBeforeWriteMsg=warning  WriteAfterWriteMsg=warning  WriteAfterReadMsg=warning  InitialValue=ones(MedusaPremixConfig.LR_out,MedusaPremixConfig.LR_in)  ShowAdditionalParam=off  OutDataTypeStr=single
  check sequence : MATLAB Function  TreatAsAtomicUnit=on
  control : MATLAB Function  TreatAsAtomicUnit=on
  process : MATLAB Function  TreatAsAtomicUnit=on
  ramping done : Outport  VectorParamsAs1DForOutWhenUnconnected=off
  wires:
  target gains (linear)/1 -> control/1(target_gains_linear)
  RTC Recv Trigger/1 -> control/Trigger
  check sequence/1(done) -> ramping done/1
  check sequence trigger/1 -> check sequence/Trigger
  ramp rate/1 -> control/2(rampRate)
  ramp time/1 -> control/3(rampTime)

== system MedusaPremix/Premix51WithMonoSurroundAndCaeWithFadeRamper/CS Processing/Mono-Surround/Left Mixer ==
  AudioIn : Inport
  MixCoeff : Inport  Port=2
  Matrix Multiply1 : Product  Multiplication=Matrix(*)
  Transpose1 : Math  Operator=transpose  SignedPower=on
  Output : Outport  VectorParamsAs1DForOutWhenUnconnected=off
  wires:
  Matrix Multiply1/1 -> Output/1
  AudioIn/1 -> Matrix Multiply1/1
  MixCoeff/1 -> Transpose1/1
  Transpose1/1 -> Matrix Multiply1/2

== system MedusaPremix/Premix51WithMonoSurroundAndCaeWithFadeRamper/CS Processing/Mono-Surround/Right Mixer ==
  AudioIn : Inport
  MixCoeff : Inport  Port=2
  Matrix Multiply1 : Product  Multiplication=Matrix(*)
  Transpose1 : Math  Operator=transpose  SignedPower=on
  Output : Outport  VectorParamsAs1DForOutWhenUnconnected=off
  wires:
  Matrix Multiply1/1 -> Output/1
  AudioIn/1 -> Matrix Multiply1/1
  MixCoeff/1 -> Transpose1/1
  Transpose1/1 -> Matrix Multiply1/2

== system MedusaPremix/Premix51WithMonoSurroundAndCaeWithFadeRamper/CS Processing/Mono-Surround/Right Mixer1 ==
  AudioIn : Inport
  MixCoeff : Inport  Port=2
  Matrix Multiply1 : Product  Multiplication=Matrix(*)
  Transpose1 : Math  Operator=transpose  SignedPower=on
  Output : Outport  VectorParamsAs1DForOutWhenUnconnected=off
  wires:
  Matrix Multiply1/1 -> Output/1
  AudioIn/1 -> Matrix Multiply1/1
  MixCoeff/1 -> Transpose1/1
  Transpose1/1 -> Matrix Multiply1/2

== system MedusaPremix/Premix51WithMonoSurroundAndCaeWithFadeRamper/CS Processing/Mono-Surround/SOS A ==
  AudioIn : Inport
  TuneIn : Inport  Port=2
  Hilbert SOS A : Subsystem  TreatAsAtomicUnit=on
  If : If  IfExpression=(u1==0) | (u1==180)
  Merge : Merge
  Pass-through : Subsystem  TreatAsAtomicUnit=on
  Out : Outport  VectorParamsAs1DForOutWhenUnconnected=off
  wires:
  AudioIn/1 -> Hilbert SOS A/1(AudioIn), Pass-through/1(In1)
  If/1 -> Pass-through/Action
  If/2 -> Hilbert SOS A/Action
  TuneIn/1 -> If/1
  Pass-through/1(Out1) -> Merge/1
  Hilbert SOS A/1(Out) -> Merge/2
  Merge/1 -> Out/1

== system MedusaPremix/Premix51WithMonoSurroundAndCaeWithFadeRamper/CS Processing/Mono-Surround/SOS B ==
  AudioIn : Inport
  TuneIn : Inport  Port=2
  Hilbert SOS B : Subsystem  TreatAsAtomicUnit=on
  If : If  IfExpression=(u1==0) | (u1==180)
  Merge : Merge
  Pass-through : Subsystem  TreatAsAtomicUnit=on
  Out : Outport  VectorParamsAs1DForOutWhenUnconnected=off
  wires:
  AudioIn/1 -> Hilbert SOS B/1(AudioIn), Pass-through/1(In1)
  If/1 -> Pass-through/Action
  If/2 -> Hilbert SOS B/Action
  TuneIn/1 -> If/1
  Pass-through/1(Out1) -> Merge/1
  Hilbert SOS B/1(Out) -> Merge/2
  Merge/1 -> Out/1

== system MedusaPremix/Premix51WithMonoSurroundAndCaeWithFadeRamper/Full Mixing Matrix_Center Surround/Fader Downmix/Fading Backward ==
  frontFadeGain : Inport
  backwardDownmixThreshold : Inport  Port=2
  backwardDownmixMax : Inport  Port=3
  Action Port : ActionPort
  Constant : Constant  OutDataTypeStr=single
  Divide : Product  Inputs=*/
  EPS : Constant  Value=eps('single')
  Max : MinMax  Function=max  Inputs=2
  Min : MinMax  Inputs=2
  Multiply : Product
  Subtract : Sum  Inputs=+-
  downmix : Outport  VectorParamsAs1DForOutWhenUnconnected=off
  wires:
  Multiply/1 -> downmix/1
  backwardDownmixMax/1 -> Multiply/2
  Subtract/1 -> Multiply/1
  Divide/1 -> Subtract/2
  Max/1 -> Divide/2
  Min/1 -> Divide/1  "minFadeGain"
  EPS/1 -> Max/2
  Constant/1 -> Subtract/1
  backwardDownmixThreshold/1 -> Max/1, Min/2
  frontFadeGain/1 -> Min/1

== system MedusaPremix/Premix51WithMonoSurroundAndCaeWithFadeRamper/Full Mixing Matrix_Center Surround/Fader Downmix/Fading Forward ==
  backFadeGain : Inport
  forwardDownmixThreshold : Inport  Port=2
  forwardDownmixMax : Inport  Port=3
  Action Port : ActionPort
  Constant : Constant  OutDataTypeStr=single
  Divide : Product  Inputs=*/
  EPS : Constant  Value=eps('single')
  Max : MinMax  Function=max  Inputs=2
  Min : MinMax  Inputs=2
  Multiply : Product
  Subtract : Sum  Inputs=+-
  downmix : Outport  VectorParamsAs1DForOutWhenUnconnected=off
  wires:
  Multiply/1 -> downmix/1
  forwardDownmixMax/1 -> Multiply/2
  Subtract/1 -> Multiply/1
  Divide/1 -> Subtract/2
  Max/1 -> Divide/2
  Min/1 -> Divide/1  "minFadeGain"
  EPS/1 -> Max/2
  Constant/1 -> Subtract/1
  forwardDownmixThreshold/1 -> Max/1, Min/2
  backFadeGain/1 -> Min/1

== system MedusaPremix/Premix51WithMonoSurroundAndCaeWithFadeRamper/Full Mixing Matrix_Left/Fader Downmix/Fading Backward ==
  frontFadeGain : Inport
  backwardDownmixThreshold : Inport  Port=2
  backwardDownmixMax : Inport  Port=3
  Action Port : ActionPort
  Constant : Constant  OutDataTypeStr=single
  Divide : Product  Inputs=*/
  EPS : Constant  Value=eps('single')
  Max : MinMax  Function=max  Inputs=2
  Min : MinMax  Inputs=2
  Multiply : Product
  Subtract : Sum  Inputs=+-
  downmix : Outport  VectorParamsAs1DForOutWhenUnconnected=off
  wires:
  Multiply/1 -> downmix/1
  backwardDownmixMax/1 -> Multiply/2
  Subtract/1 -> Multiply/1
  Divide/1 -> Subtract/2
  Max/1 -> Divide/2
  Min/1 -> Divide/1  "minFadeGain"
  EPS/1 -> Max/2
  Constant/1 -> Subtract/1
  backwardDownmixThreshold/1 -> Max/1, Min/2
  frontFadeGain/1 -> Min/1

== system MedusaPremix/Premix51WithMonoSurroundAndCaeWithFadeRamper/Full Mixing Matrix_Left/Fader Downmix/Fading Forward ==
  backFadeGain : Inport
  forwardDownmixThreshold : Inport  Port=2
  forwardDownmixMax : Inport  Port=3
  Action Port : ActionPort
  Constant : Constant  OutDataTypeStr=single
  Divide : Product  Inputs=*/
  EPS : Constant  Value=eps('single')
  Max : MinMax  Function=max  Inputs=2
  Min : MinMax  Inputs=2
  Multiply : Product
  Subtract : Sum  Inputs=+-
  downmix : Outport  VectorParamsAs1DForOutWhenUnconnected=off
  wires:
  Multiply/1 -> downmix/1
  forwardDownmixMax/1 -> Multiply/2
  Subtract/1 -> Multiply/1
  Divide/1 -> Subtract/2
  Max/1 -> Divide/2
  Min/1 -> Divide/1  "minFadeGain"
  EPS/1 -> Max/2
  Constant/1 -> Subtract/1
  forwardDownmixThreshold/1 -> Max/1, Min/2
  backFadeGain/1 -> Min/1

== system MedusaPremix/Premix51WithMonoSurroundAndCaeWithFadeRamper/Full Mixing Matrix_Right/Fader Downmix/Fading Backward ==
  frontFadeGain : Inport
  backwardDownmixThreshold : Inport  Port=2
  backwardDownmixMax : Inport  Port=3
  Action Port : ActionPort
  Constant : Constant  OutDataTypeStr=single
  Divide : Product  Inputs=*/
  EPS : Constant  Value=eps('single')
  Max : MinMax  Function=max  Inputs=2
  Min : MinMax  Inputs=2
  Multiply : Product
  Subtract : Sum  Inputs=+-
  downmix : Outport  VectorParamsAs1DForOutWhenUnconnected=off
  wires:
  Multiply/1 -> downmix/1
  backwardDownmixMax/1 -> Multiply/2
  Subtract/1 -> Multiply/1
  Divide/1 -> Subtract/2
  Max/1 -> Divide/2
  Min/1 -> Divide/1  "minFadeGain"
  EPS/1 -> Max/2
  Constant/1 -> Subtract/1
  backwardDownmixThreshold/1 -> Max/1, Min/2
  frontFadeGain/1 -> Min/1

== system MedusaPremix/Premix51WithMonoSurroundAndCaeWithFadeRamper/Full Mixing Matrix_Right/Fader Downmix/Fading Forward ==
  backFadeGain : Inport
  forwardDownmixThreshold : Inport  Port=2
  forwardDownmixMax : Inport  Port=3
  Action Port : ActionPort
  Constant : Constant  OutDataTypeStr=single
  Divide : Product  Inputs=*/
  EPS : Constant  Value=eps('single')
  Max : MinMax  Function=max  Inputs=2
  Min : MinMax  Inputs=2
  Multiply : Product
  Subtract : Sum  Inputs=+-
  downmix : Outport  VectorParamsAs1DForOutWhenUnconnected=off
  wires:
  Multiply/1 -> downmix/1
  forwardDownmixMax/1 -> Multiply/2
  Subtract/1 -> Multiply/1
  Divide/1 -> Subtract/2
  Max/1 -> Divide/2
  Min/1 -> Divide/1  "minFadeGain"
  EPS/1 -> Max/2
  Constant/1 -> Subtract/1
  forwardDownmixThreshold/1 -> Max/1, Min/2
  backFadeGain/1 -> Min/1

== system MedusaPremix/PremixWithMonoSurround/CS Processing/Mono-Surround/Left Mixer ==
  AudioIn : Inport
  MixCoeff : Inport  Port=2
  Matrix Multiply1 : Product  Multiplication=Matrix(*)
  Transpose1 : Math  Operator=transpose  SignedPower=on
  Output : Outport  VectorParamsAs1DForOutWhenUnconnected=off
  wires:
  Matrix Multiply1/1 -> Output/1
  AudioIn/1 -> Matrix Multiply1/1
  MixCoeff/1 -> Transpose1/1
  Transpose1/1 -> Matrix Multiply1/2

== system MedusaPremix/PremixWithMonoSurround/CS Processing/Mono-Surround/MS Tune ==
  TOP : TOP/TOP  TriggerInit=[260 -150 405 -90]  TopName=Phi  DataType=single  BankNumber=0  Role=Automatic
      settings: SourceProductName=Bose Talaria
  TOP1 : TOP/TOP  TriggerInit=[260 -70 405 -10]  TopName=CosPhi  DataType=single  BankNumber=0  Role=Automatic
      settings: SourceProductName=Bose Talaria
  TOP2 : TOP/TOP  TriggerInit=[260 10 405 70]  TopName=SinPhi  DataType=single  BankNumber=0  Role=Automatic
      settings: SourceProductName=Bose Talaria
  TranslateTrigger : TuneVar/TranslateTrigger  TriggerInit=[66 -245 104 -190]
      settings: SourceProductName=Bose Talaria
  Tune Variable : TuneVar/Tune Variable  TuneName=PhaseAngle  SpecifyMaxSize=off  VariableDim=1 (Row)  MaxSize=[1 1]  PackageName=mode  TunabilityNumber=1  MinValue=[]  MaxValue=[]  TriggerInit=[-270 -65 -100 -15]  MaskValue=MSConfig.DefaultPhaseAngle
      settings: SourceProductName=Bose Talaria
  translation : MATLAB Function  TreatAsAtomicUnit=on
  phi : Outport  VectorParamsAs1DForOutWhenUnconnected=off
  cos(phi) : Outport  Port=2  VectorParamsAs1DForOutWhenUnconnected=off
  sin(phi) : Outport  Port=3  VectorParamsAs1DForOutWhenUnconnected=off
  wires:
  translation/1(phi) -> TOP/1
  TranslateTrigger/1 -> translation/Trigger
  TOP/1 -> phi/1  "Phi"
  Tune Variable/1 -> translation/1(PhaseAngle)  "PhaseAngle"
  translation/2(cos_phi) -> TOP1/1
  TOP1/1 -> cos(phi)/1  "CosPhi"
  translation/3(sin_phi) -> TOP2/1
  TOP2/1 -> sin(phi)/1  "SinPhi"

== system MedusaPremix/PremixWithMonoSurround/CS Processing/Mono-Surround/Right Mixer ==
  AudioIn : Inport
  MixCoeff : Inport  Port=2
  Matrix Multiply1 : Product  Multiplication=Matrix(*)
  Transpose1 : Math  Operator=transpose  SignedPower=on
  Output : Outport  VectorParamsAs1DForOutWhenUnconnected=off
  wires:
  Matrix Multiply1/1 -> Output/1
  AudioIn/1 -> Matrix Multiply1/1
  MixCoeff/1 -> Transpose1/1
  Transpose1/1 -> Matrix Multiply1/2

== system MedusaPremix/PremixWithMonoSurround/CS Processing/Mono-Surround/SOS A ==
  AudioIn : Inport
  TuneIn : Inport  Port=2
  Hilbert SOS A : Subsystem  TreatAsAtomicUnit=on
  If : If  IfExpression=(u1==0) | (u1==180)
  Merge : Merge
  Pass-through : Subsystem  TreatAsAtomicUnit=on
  Out : Outport  VectorParamsAs1DForOutWhenUnconnected=off
  wires:
  AudioIn/1 -> Hilbert SOS A/1(AudioIn), Pass-through/1(In1)
  If/1 -> Pass-through/Action
  If/2 -> Hilbert SOS A/Action
  TuneIn/1 -> If/1
  Pass-through/1(Out1) -> Merge/1
  Hilbert SOS A/1(Out) -> Merge/2
  Merge/1 -> Out/1

== system MedusaPremix/PremixWithMonoSurround/CS Processing/Mono-Surround/SOS B ==
  AudioIn : Inport
  TuneIn : Inport  Port=2
  Hilbert SOS B : Subsystem  TreatAsAtomicUnit=on
  If : If  IfExpression=(u1==0) | (u1==180)
  Merge : Merge
  Pass-through : Subsystem  TreatAsAtomicUnit=on
  Out : Outport  VectorParamsAs1DForOutWhenUnconnected=off
  wires:
  AudioIn/1 -> Hilbert SOS B/1(AudioIn), Pass-through/1(In1)
  If/1 -> Pass-through/Action
  If/2 -> Hilbert SOS B/Action
  TuneIn/1 -> If/1
  Pass-through/1(Out1) -> Merge/1
  Hilbert SOS B/1(Out) -> Merge/2
  Merge/1 -> Out/1

== system MedusaPremix/PremixWithMonoSurround/Full Mixing Matrix_Center Surround/Fader Downmix/Fading Backward ==
  frontFadeGain : Inport
  backwardDownmixThreshold : Inport  Port=2
  backwardDownmixMax : Inport  Port=3
  Action Port : ActionPort
  Constant : Constant  OutDataTypeStr=single
  Divide : Product  Inputs=*/
  EPS : Constant  Value=eps('single')
  Max : MinMax  Function=max  Inputs=2
  Min : MinMax  Inputs=2
  Multiply : Product
  Subtract : Sum  Inputs=+-
  downmix : Outport  VectorParamsAs1DForOutWhenUnconnected=off
  wires:
  Multiply/1 -> downmix/1
  backwardDownmixMax/1 -> Multiply/2
  Subtract/1 -> Multiply/1
  Divide/1 -> Subtract/2
  Max/1 -> Divide/2
  Min/1 -> Divide/1  "minFadeGain"
  EPS/1 -> Max/2
  Constant/1 -> Subtract/1
  backwardDownmixThreshold/1 -> Max/1, Min/2
  frontFadeGain/1 -> Min/1

== system MedusaPremix/PremixWithMonoSurround/Full Mixing Matrix_Center Surround/Fader Downmix/Fading Forward ==
  backFadeGain : Inport
  forwardDownmixThreshold : Inport  Port=2
  forwardDownmixMax : Inport  Port=3
  Action Port : ActionPort
  Constant : Constant  OutDataTypeStr=single
  Divide : Product  Inputs=*/
  EPS : Constant  Value=eps('single')
  Max : MinMax  Function=max  Inputs=2
  Min : MinMax  Inputs=2
  Multiply : Product
  Subtract : Sum  Inputs=+-
  downmix : Outport  VectorParamsAs1DForOutWhenUnconnected=off
  wires:
  Multiply/1 -> downmix/1
  forwardDownmixMax/1 -> Multiply/2
  Subtract/1 -> Multiply/1
  Divide/1 -> Subtract/2
  Max/1 -> Divide/2
  Min/1 -> Divide/1  "minFadeGain"
  EPS/1 -> Max/2
  Constant/1 -> Subtract/1
  forwardDownmixThreshold/1 -> Max/1, Min/2
  backFadeGain/1 -> Min/1
